simulink model "chalgyafzintegrationkrrhe"  (R2024b)
settings: Solver=ode4  StartTime=0.0  StopTime=150  FixedStep=0.001  RelTol=1e-3
values from neighbouring files (symbols this model uses):
  kappa = (dx .* d2y - dy .* d2x) ./          ((dx.^2 + dy.^2).^(3/2) + 1e-6)    [Buildmadrasspeedway.m]
  pathX = ppval(ppx,s)    [Buildmadrasspeedway.m]
  pathY = ppval(ppy,s)    [Buildmadrasspeedway.m]
  pathYaw = unwrap(atan2(dy,dx))    [Buildmadrasspeedway.m]
  s = 0:ds:t(end)    [Buildmadrasspeedway.m]
undefined symbols (not defined in the file or in its folder): v_ref
libraries: autolibsharedcoupling x1, vehdynlibsteering x1, autolibmappedmotor x1, vehdynlibdriver x1, autolibshared x1
(part 2 of 2)

== matlab function chalgyafzintegrationkrrhe/MATLAB Function8 ==
  settings: updateMethod=DISCRETE
  data: X input; LongRef output; Y input; Vx input; pathX input; pathY input; pathYaw input; v_ref input; LatRef output; YawRef output; VelRef output; CurvRef output; kappa input
function [LongRef, LatRef, YawRef, VelRef, CurvRef] = ...
    PathRefGenerator(X, Y, Vx, pathX, pathY, pathYaw, v_ref, kappa)

%#codegen

persistent lastIdx

N = length(pathX);

%% ============================================================
% INITIALIZATION
% =============================================================

if N < 2
    LongRef = X;
    LatRef  = Y;
    YawRef  = 0;
    VelRef  = 0;
    CurvRef = 0;
    return;
end

if isempty(lastIdx)

    minDistSq = 1e12;
    lastIdx = 1;

    for k = 1:N

        dx = X - pathX(k);
        dy = Y - pathY(k);

        d2 = dx*dx + dy*dy;

        if d2 < minDistSq
            minDistSq = d2;
            lastIdx = k;
        end
    end
end

%% ============================================================
% 1. FIND CLOSEST PATH POINT
% =============================================================

backwardWindow = 20;
forwardWindow  = 100;

minDistSq = 1e12;
bestIdx = lastIdx;

for i = -backwardWindow:forwardWindow

    k = lastIdx + i;

    while k > N
        k = k - N;
    end

    while k < 1
        k = k + N;
    end

    dx = X - pathX(k);
    dy = Y - pathY(k);

    d2 = dx*dx + dy*dy;

    if d2 < minDistSq
        minDistSq = d2;
        bestIdx = k;
    end
end

%% ============================================================
% 2. LOST VEHICLE RECOVERY
% =============================================================

if minDistSq > 30*30

    globalMinDistSq = 1e12;
    globalBestIdx = bestIdx;

    for k = 1:N

        dx = X - pathX(k);
        dy = Y - pathY(k);

        d2 = dx*dx + dy*dy;

        if d2 < globalMinDistSq
            globalMinDistSq = d2;
            globalBestIdx = k;
        end
    end

    bestIdx = globalBestIdx;
end

lastIdx = bestIdx;

%% ============================================================
% 3. STEERING LOOKAHEAD
% =============================================================

Vforward = max(Vx,0);

lookaheadDist = 8 + 0.40*Vforward;

if lookaheadDist < 8
    lookaheadDist = 8;
end

if lookaheadDist > 25
    lookaheadDist = 25;
end

%% ============================================================
% 4. FIND STEERING TARGET USING DISTANCE
% =============================================================

steerIdx = lastIdx;

distanceTravelled = 0;

while distanceTravelled < lookaheadDist

    nextIdx = steerIdx + 1;

    if nextIdx > N
        nextIdx = 1;
    end

    dx = pathX(nextIdx) - pathX(steerIdx);
    dy = pathY(nextIdx) - pathY(steerIdx);

    segmentLength = hypot(dx,dy);

    if segmentLength < 1e-4
        segmentLength = 1e-4;
    end

    distanceTravelled = distanceTravelled + segmentLength;

    steerIdx = nextIdx;

    if steerIdx == lastIdx
        break;
    end
end

%% ============================================================
% 5. STEERING REFERENCES
% =============================================================

LongRef = pathX(steerIdx);
LatRef  = pathY(steerIdx);

%% Yaw from path geometry

nextIdx = steerIdx + 1;

if nextIdx > N
    nextIdx = 1;
end

dx = pathX(nextIdx) - pathX(steerIdx);
dy = pathY(nextIdx) - pathY(steerIdx);

if hypot(dx,dy) > 1e-4
    YawRef = atan2(dy,dx);
else
    YawRef = pathYaw(steerIdx);
end

%% ============================================================
% 6. CURVATURE
% =============================================================

CurvRef = kappa(steerIdx);

%% ============================================================
% 7. SPEED PREVIEW
% =============================================================
%
% DO NOT simply use v_ref(steerIdx).
%
% Look ahead along the track and find the minimum speed
% requirement over a preview distance.

speedPreviewDist = 40.0;

speedIdx = lastIdx;

distanceTravelled = 0;

VelRef = v_ref(lastIdx);

while distanceTravelled < speedPreviewDist

    nextIdx = speedIdx + 1;

    if nextIdx > N
        nextIdx = 1;
    end

    dx = pathX(nextIdx) - pathX(speedIdx);
    dy = pathY(nextIdx) - pathY(speedIdx);

    segmentLength = hypot(dx,dy);

    if segmentLength < 1e-4
        segmentLength = 1e-4;
    end

    distanceTravelled = distanceTravelled + segmentLength;

    speedIdx = nextIdx;

    if v_ref(speedIdx) < VelRef
        VelRef = v_ref(speedIdx);
    end

    if speedIdx == lastIdx
        break;
    end
end

%% ============================================================
% 8. PREVENT EXTREME SPEED REFERENCE
% =============================================================

if VelRef < 5.0
    VelRef = 5.0;
end

end

== matlab function chalgyafzintegrationkrrhe/Rear_left tire  ==
  data: alpha input; Fx output; gamma input; kappa input; Fz input; Vc input; a input; b input; re input; mu0 input; cp input; n input; Fy output; Mz output; Mx output; slide_count output
function [Fx,Fy,Mz,Mx,slide_count] = tread_model( ...
                alpha,...
                gamma,...
                kappa,...
                Fz,...
                Vc,...
                a,b,re,...
                mu0,...
                cp,...
                n)

%%%%%%%%%%%%%%%%%%%%%%%%%%%%%%%%%%%%%%%%%%%%%%%%%%%%%%%%%%%%
% CONTACT PATCH
%%%%%%%%%%%%%%%%%%%%%%%%%%%%%%%%%%%%%%%%%%%%%%%%%%%%%%%%%%%%

xb = linspace(a,-a,n);

dx = abs(xb(2)-xb(1));

%%%%%%%%%%%%%%%%%%%%%%%%%%%%%%%%%%%%%%%%%%%%%%%%%%%%%%%%%%%%
% ROLLING KINEMATICS
%%%%%%%%%%%%%%%%%%%%%%%%%%%%%%%%%%%%%%%%%%%%%%%%%%%%%%%%%%%%

Vr = Vc/(1-kappa);

Omega = Vr/re;

dt = dx/Vr;

%%%%%%%%%%%%%%%%%%%%%%%%%%%%%%%%%%%%%%%%%%%%%%%%%%%%%%%%%%%%
% SLIP VELOCITIES
%%%%%%%%%%%%%%%%%%%%%%%%%%%%%%%%%%%%%%%%%%%%%%%%%%%%%%%%%%%%

Vsx = -Vc*kappa;

Vsy = -Vc*tan(alpha);

%%%%%%%%%%%%%%%%%%%%%%%%%%%%%%%%%%%%%%%%%%%%%%%%%%%%%%%%%%%%
% MULTI ROW TREAD
%%%%%%%%%%%%%%%%%%%%%%%%%%%%%%%%%%%%%%%%%%%%%%%%%%%%%%%%%%%%

nRows = 11;

yrow = linspace(-b,b,nRows);

dyrow = (2*b)/(nRows-1);

%%%%%%%%%%%%%%%%%%%%%%%%%%%%%%%%%%%%%%%%%%%%%%%%%%%%%%%%%%%%
% OUTPUT INITIALIZATION
%%%%%%%%%%%%%%%%%%%%%%%%%%%%%%%%%%%%%%%%%%%%%%%%%%%%%%%%%%%%

Fx = 0;
Fy = 0;
Mz = 0;
Mx = 0;

slide_count = 0;

%%%%%%%%%%%%%%%%%%%%%%%%%%%%%%%%%%%%%%%%%%%%%%%%%%%%%%%%%%%%
% PRESSURE NORMALIZATION
%%%%%%%%%%%%%%%%%%%%%%%%%%%%%%%%%%%%%%%%%%%%%%%%%%%%%%%%%%%%

ShapeSum = 0;

for r = 1:nRows

    yb0 = yrow(r);

    for i = 1:n

        px = max(0,1-(xb(i)/a)^2);

        py = sqrt(max(0,1-(yb0/b)^2));

        ShapeSum = ShapeSum + px*py*dx*dyrow;

    end
end

qz0 = Fz/ShapeSum;

%%%%%%%%%%%%%%%%%%%%%%%%%%%%%%%%%%%%%%%%%%%%%%%%%%%%%%%%%%%%
% MAIN LOOP
%%%%%%%%%%%%%%%%%%%%%%%%%%%%%%%%%%%%%%%%%%%%%%%%%%%%%%%%%%%%

for r = 1:nRows

    yb0 = yrow(r);

    ex = 0;
    ey = 0;

    for i = 1:n

        px = max(0,1-(xb(i)/a)^2);

        py = sqrt(max(0,1-(yb0/b)^2));

        qz = qz0*px*py;

        if qz <= 0
            continue
        end

        dybdx = (xb(i)/re)*sin(gamma);

        Vbx = Vsx + yb0*Omega*sin(gamma);

        Vby = Vsy - Vr*dybdx;

        %%%%%%%%%%%%%%%%%%%%%%%%%%%%%%%%%%%%%%%%%%%%%%%%%%%%
        % CONSTANT FRICTION
        %%%%%%%%%%%%%%%%%%%%%%%%%%%%%%%%%%%%%%%%%%%%%%%%%%%%

        qlimit = mu0*qz;

        Dsx = Vbx*dt;

        Dsy = Vby*dt;

        ex_trial = ex - Dsx;

        ey_trial = ey - Dsy;

        qx_trial = cp*ex_trial;

        qy_trial = cp*ey_trial;

        qtrial = hypot(qx_trial,qy_trial);

        %%%%%%%%%%%%%%%%%%%%%%%%%%%%%%%%%%%%%%%%%%%%%%%%%%%%
        % ADHESION
        %%%%%%%%%%%%%%%%%%%%%%%%%%%%%%%%%%%%%%%%%%%%%%%%%%%%

        if qtrial <= qlimit

            ex = ex_trial;
            ey = ey_trial;

            qx = cp*ex;
            qy = cp*ey;

        %%%%%%%%%%%%%%%%%%%%%%%%%%%%%%%%%%%%%%%%%%%%%%%%%%%%
        % SLIDING
        %%%%%%%%%%%%%%%%%%%%%%%%%%%%%%%%%%%%%%%%%%%%%%%%%%%%

        else

            slide_count = slide_count + 1;

            e_i = qlimit/cp;

            norm_trial = hypot(ex_trial,ey_trial);

            if norm_trial > 1e-12

                ex = e_i*ex_trial/norm_trial;

                ey = e_i*ey_trial/norm_trial;

            else

                ex = 0;
                ey = 0;

            end

            qx = cp*ex;
            qy = cp*ey;

        end

        dA = dx*dyrow;

        dFx = qx*dA;
        dFy = qy*dA;

        Fx = Fx + dFx;
        Fy = Fy + dFy;

        Mz = Mz + xb(i)*dFy - yb0*dFx;

        Mx = Mx + yb0*dFy;

    end
end

end

== matlab function chalgyafzintegrationkrrhe/MATLAB Function9 ==
  data: X input; stop output; Y input; pathX1 input; pathY1 input; t input
function stop = LapDetector(X, Y, pathX1, pathY1, t)
%#codegen
    dist = hypot(X - pathX1, Y - pathY1);
    
    % Only trigger after 30 seconds (to avoid stopping at t=0 start point)
    % and when within 10 meters of start/finish line
    if (t > 30) && (dist < 10)
        stop = 1;   % Non-zero triggers Stop Simulation block
    else
        stop = 0;
    end
end

== matlab function chalgyafzintegrationkrrhe/MATLAB Function10 ==
  data: xdot input; ax_G output; ydot input; r input; xdot_deriv input; ydot_deriv input; ay_G output
function [ax_G, ay_G] = calculate_GG(xdot, ydot, r, xdot_deriv, ydot_deriv)
    % Define gravity
    g = 9.80665; % m/s^2
    
    % Calculate true body-frame accelerations (m/s^2)
    % Accounting for centripetal acceleration (v * r)
    ax_mps2 = xdot_deriv - (ydot * r);
    ay_mps2 = ydot_deriv + (xdot * r);
    
    % Convert to G-Forces
    ax_G = ax_mps2 / g;
    ay_G = ay_mps2 / g;
end

== matlab function chalgyafzintegrationkrrhe/VehicleVelocityDerivative ==
  settings: updateMethod=DISCRETE
  data: Ux input; Ux_dot output; Uy input; Uy_dot output
function [Ux_dot, Uy_dot] = VehicleVelocityDerivative(Ux, Uy)
%#codegen
%
% Discrete second-order backward derivative.
%
% Block sample time must be fixed at Ts = 0.01 s.
%
% Ux     : longitudinal body velocity [m/s]
% Uy     : lateral body velocity [m/s]
%
% Ux_dot : dUx/dt [m/s^2]
% Uy_dot : dUy/dt [m/s^2]

persistent Ux_1 Ux_2
persistent Uy_1 Uy_2
persistent initialized

Ts = 0.001;

if isempty(initialized)

    % Initialize history with the actual initial velocities.
    Ux_1 = Ux;
    Ux_2 = Ux;

    Uy_1 = Uy;
    Uy_2 = Uy;

    initialized = true;

    Ux_dot = 0;
    Uy_dot = 0;

    return;
end

% Second-order backward difference
Ux_dot = ...
    (3*Ux - 4*Ux_1 + Ux_2)/(2*Ts);

Uy_dot = ...
    (3*Uy - 4*Uy_1 + Uy_2)/(2*Ts);

% Update history
Ux_2 = Ux_1;
Ux_1 = Ux;

Uy_2 = Uy_1;
Uy_1 = Uy;

end

== matlab function chalgyafzintegrationkrrhe/Wheel kinematics ==
  data: Ux input; alphaFL output; Uy input; r input; deltaFL input; deltaFR input; omegaFL input; omegaFR input; omegaRL input; omegaRR input; lf input; lr input; tf input; tr input; Rw input; alphaFR output; alphaRL output; alphaRR output; kappaFL output; kappaFR output; kappaRL output; kappaRR output; VcFL output; VcFR output; VcRL output; VcRR output
function [alphaFL,alphaFR,alphaRL,alphaRR, ...
          kappaFL,kappaFR,kappaRL,kappaRR, ...
          VcFL,VcFR,VcRL,VcRR] = WheelKinematics( ...
          Ux,Uy,r, ...
          deltaFL,deltaFR, ...
          omegaFL,omegaFR,omegaRL,omegaRR, ...
          lf,lr,tf,tr,Rw)
%#codegen

%% =========================================================
% Numerical protection
%% =========================================================

Veps = 0.5;

%% =========================================================
% Wheel centre velocities in vehicle frame
% x positive forward, y positive left, yaw rate r positive CCW
%% =========================================================

VxFL = Ux - r*tf/2;
VyFL = Uy + r*lf;

VxFR = Ux + r*tf/2;
VyFR = Uy + r*lf;

VxRL = Ux - r*tr/2;
VyRL = Uy - r*lr;

VxRR = Ux + r*tr/2;
VyRR = Uy - r*lr;

%% =========================================================
% Transform front wheel velocities into wheel frame
%% =========================================================

VxwFL =  VxFL*cos(deltaFL) + VyFL*sin(deltaFL);
VywFL = -VxFL*sin(deltaFL) + VyFL*cos(deltaFL);

VxwFR =  VxFR*cos(deltaFR) + VyFR*sin(deltaFR);
VywFR = -VxFR*sin(deltaFR) + VyFR*cos(deltaFR);

%% =========================================================
% Rear wheels are not steered
%% =========================================================

VxwRL = VxRL;
VywRL = VyRL;

VxwRR = VxRR;
VywRR = VyRR;

%% =========================================================
% Slip angle convention for your tire model
%
% Important:
% Your tire model gives positive Fy for positive alpha.
% So we use:
%
% alpha = -atan2(Vyw,Vxw)
%
% This makes positive steering produce positive tire lateral force.
%% =========================================================

alphaFL = -atan2(VywFL, max(abs(VxwFL),Veps));
alphaFR = -atan2(VywFR, max(abs(VxwFR),Veps));
alphaRL = -atan2(VywRL, max(abs(VxwRL),Veps));
alphaRR = -atan2(VywRR, max(abs(VxwRR),Veps));

%% =========================================================
% Longitudinal contact velocity for tire model
%% =========================================================

VcFL = max(abs(VxwFL),Veps);
VcFR = max(abs(VxwFR),Veps);
VcRL = max(abs(VxwRL),Veps);
VcRR = max(abs(VxwRR),Veps);

%% =========================================================
% Slip ratio
%
% Positive kappa = driving
% Negative kappa = braking
%% =========================================================

kappaFL = (Rw*omegaFL - VxwFL)/max(abs(VxwFL),Veps);
kappaFR = (Rw*omegaFR - VxwFR)/max(abs(VxwFR),Veps);
kappaRL = (Rw*omegaRL - VxwRL)/max(abs(VxwRL),Veps);
kappaRR = (Rw*omegaRR - VxwRR)/max(abs(VxwRR),Veps);

%% =========================================================
% Saturation to protect tire model
%% =========================================================

kappaFL = min(max(kappaFL,-0.80),0.80);
kappaFR = min(max(kappaFR,-0.80),0.80);
kappaRL = min(max(kappaRL,-0.80),0.80);
kappaRR = min(max(kappaRR,-0.80),0.80);

end

== matlab function chalgyafzintegrationkrrhe/Front_Left_tire ==
  data: alpha input; Fx output; gamma input; kappa input; Fz input; Vc input; a input; b input; re input; mu0 input; cp input; n input; Fy output; Mz output; Mx output; slide_count output
function [Fx,Fy,Mz,Mx,slide_count] = tread_model( ...
                alpha,...
                gamma,...
                kappa,...
                Fz,...
                Vc,...
                a,b,re,...
                mu0,...
                cp,...
                n)

%%%%%%%%%%%%%%%%%%%%%%%%%%%%%%%%%%%%%%%%%%%%%%%%%%%%%%%%%%%%
% CONTACT PATCH
%%%%%%%%%%%%%%%%%%%%%%%%%%%%%%%%%%%%%%%%%%%%%%%%%%%%%%%%%%%%

xb = linspace(a,-a,n);

dx = abs(xb(2)-xb(1));

%%%%%%%%%%%%%%%%%%%%%%%%%%%%%%%%%%%%%%%%%%%%%%%%%%%%%%%%%%%%
% ROLLING KINEMATICS
%%%%%%%%%%%%%%%%%%%%%%%%%%%%%%%%%%%%%%%%%%%%%%%%%%%%%%%%%%%%

Vr = Vc/(1-kappa);

Omega = Vr/re;

dt = dx/Vr;

%%%%%%%%%%%%%%%%%%%%%%%%%%%%%%%%%%%%%%%%%%%%%%%%%%%%%%%%%%%%
% SLIP VELOCITIES
%%%%%%%%%%%%%%%%%%%%%%%%%%%%%%%%%%%%%%%%%%%%%%%%%%%%%%%%%%%%

Vsx = -Vc*kappa;

Vsy = -Vc*tan(alpha);

%%%%%%%%%%%%%%%%%%%%%%%%%%%%%%%%%%%%%%%%%%%%%%%%%%%%%%%%%%%%
% MULTI ROW TREAD
%%%%%%%%%%%%%%%%%%%%%%%%%%%%%%%%%%%%%%%%%%%%%%%%%%%%%%%%%%%%

nRows = 11;

yrow = linspace(-b,b,nRows);

dyrow = (2*b)/(nRows-1);

%%%%%%%%%%%%%%%%%%%%%%%%%%%%%%%%%%%%%%%%%%%%%%%%%%%%%%%%%%%%
% OUTPUT INITIALIZATION
%%%%%%%%%%%%%%%%%%%%%%%%%%%%%%%%%%%%%%%%%%%%%%%%%%%%%%%%%%%%

Fx = 0;
Fy = 0;
Mz = 0;
Mx = 0;

slide_count = 0;

%%%%%%%%%%%%%%%%%%%%%%%%%%%%%%%%%%%%%%%%%%%%%%%%%%%%%%%%%%%%
% PRESSURE NORMALIZATION
%%%%%%%%%%%%%%%%%%%%%%%%%%%%%%%%%%%%%%%%%%%%%%%%%%%%%%%%%%%%

ShapeSum = 0;

for r = 1:nRows

    yb0 = yrow(r);

    for i = 1:n

        px = max(0,1-(xb(i)/a)^2);

        py = sqrt(max(0,1-(yb0/b)^2));

        ShapeSum = ShapeSum + px*py*dx*dyrow;

    end
end

qz0 = Fz/ShapeSum;

%%%%%%%%%%%%%%%%%%%%%%%%%%%%%%%%%%%%%%%%%%%%%%%%%%%%%%%%%%%%
% MAIN LOOP
%%%%%%%%%%%%%%%%%%%%%%%%%%%%%%%%%%%%%%%%%%%%%%%%%%%%%%%%%%%%

for r = 1:nRows

    yb0 = yrow(r);

    ex = 0;
    ey = 0;

    for i = 1:n

        px = max(0,1-(xb(i)/a)^2);

        py = sqrt(max(0,1-(yb0/b)^2));

        qz = qz0*px*py;

        if qz <= 0
            continue
        end

        dybdx = (xb(i)/re)*sin(gamma);

        Vbx = Vsx + yb0*Omega*sin(gamma);

        Vby = Vsy - Vr*dybdx;

        %%%%%%%%%%%%%%%%%%%%%%%%%%%%%%%%%%%%%%%%%%%%%%%%%%%%
        % CONSTANT FRICTION
        %%%%%%%%%%%%%%%%%%%%%%%%%%%%%%%%%%%%%%%%%%%%%%%%%%%%

        qlimit = mu0*qz;

        Dsx = Vbx*dt;

        Dsy = Vby*dt;

        ex_trial = ex - Dsx;

        ey_trial = ey - Dsy;

        qx_trial = cp*ex_trial;

        qy_trial = cp*ey_trial;

        qtrial = hypot(qx_trial,qy_trial);

        %%%%%%%%%%%%%%%%%%%%%%%%%%%%%%%%%%%%%%%%%%%%%%%%%%%%
        % ADHESION
        %%%%%%%%%%%%%%%%%%%%%%%%%%%%%%%%%%%%%%%%%%%%%%%%%%%%

        if qtrial <= qlimit

            ex = ex_trial;
            ey = ey_trial;

            qx = cp*ex;
            qy = cp*ey;

        %%%%%%%%%%%%%%%%%%%%%%%%%%%%%%%%%%%%%%%%%%%%%%%%%%%%
        % SLIDING
        %%%%%%%%%%%%%%%%%%%%%%%%%%%%%%%%%%%%%%%%%%%%%%%%%%%%

        else

            slide_count = slide_count + 1;

            e_i = qlimit/cp;

            norm_trial = hypot(ex_trial,ey_trial);

            if norm_trial > 1e-12

                ex = e_i*ex_trial/norm_trial;

                ey = e_i*ey_trial/norm_trial;

            else

                ex = 0;
                ey = 0;

            end

            qx = cp*ex;
            qy = cp*ey;

        end

        dA = dx*dyrow;

        dFx = qx*dA;
        dFy = qy*dA;

        Fx = Fx + dFx;
        Fy = Fy + dFy;

        Mz = Mz + xb(i)*dFy - yb0*dFx;

        Mx = Mx + yb0*dFy;

    end
end

end
